simulink model "DPWM_VMC_lec22_r2017b"  (R2017b)
settings: Solver=FixedStepAuto  StartTime=0.0  StopTime=3e-3  FixedStep=Ts  RelTol=1e-3
PostLoadFcn:
  | , if any(exist('dsrtsu_mdlpostloadfcn', 'file') == [2, 3, 6]), try dsrtsu_mdlpostloadfcn('Execute', bdroot); catch fprintf('Error in PostLoadFcn (dsrtsu_mdlpostloadfcn) for model "%s":\n %s\n', bdroot, lasterr); end, end,
  | init_practical_voltage_source;
  | init_parameters;
InitFcn:
  | init_practical_voltage_source;
  | init_parameters;
values from neighbouring files (symbols this model uses):
  C = 200e-6    (= 0.0002)    [init_parameters.m]
  DCM_en = 0    [init_parameters.m]
  I0_final = 20    [init_parameters.m]
  I0_stepTime = 2.0e-3    (= 0.002)    [init_parameters.m]
  i_L_init = 1    [init_parameters.m]
  Kd = 0.5*C    (= 0.0001)    [init_parameters.m]
  Ki = 50000    [init_parameters.m]
  Kp = 10    [init_parameters.m]
  L = 0.5e-6    (= 5e-07)    [init_parameters.m]
  N = 1000    [init_parameters.m]
  R = 1    [init_parameters.m]
  r_C = 3e-3    (= 0.003)    [init_parameters.m]
  r_d = rds_on_sw2    (= 0.005)    [init_parameters.m]
  r_L = 5e-3    (= 0.005)    [init_parameters.m]
  rds_on_sw1 = 5e-3    (= 0.005)    [init_parameters.m]
  T_Vin_stepTime = 1.5e-3    (= 0.0015)    [init_parameters.m]
  Ts = 10e-9    (= 1e-08)    [init_parameters.m]
  Tsw = 2e-6    (= 2e-06)    [init_parameters.m]
  v_C_init = 1.1    [init_parameters.m]
  Vd = 0.55    [init_parameters.m]
  Vff = 1/Vin    (= 0.0833333333333)    [init_parameters.m]
  Vin = 12    [init_parameters.m]
  Vin_final = 0    [init_parameters.m]
  Vmax = 10    [init_parameters.m]
  Vref = 1.0    (= 1)    [init_parameters.m]
  Vref_final = 0    [init_parameters.m]
  Vref_stepTime = 2.2e-3    (= 0.0022)    [init_parameters.m]
libraries: simulink x5
Description:
  | Standard RTI1005 template.
  | Supported MATLAB version:  R2017b.
settings Model: Tag=RTI1005  DSRTSU_INTERNAL_RTI_VER=540  DSRTSU_INTERNAL_RTI_TYPE=rti1005  RTICANMMDATA=struct('GeneralSetupData',struct('modelroot','C:\Projects\Simulink\PE_2\w1\lec7','generalsettings',struct('filesettings',struct('destfolder',struct('Name','RTICANMM_FILES','Check',1),'buildfolder',struct('Name','.','Check',1),'AbsDestfolder',struct('Name','C:\Projects\Simulink\PE_2\w1\lec7\RTICANMM_FILES'),'AbsBuildfolder',struct('Name','C:\Projects\Simulink\PE_2\w1\lec7'))),'options',struct('addpaths',1,'rmpaths',1,'addtrcexclusion',logical(1),'cannavigator',struct('checkmonitoring',0),'show_usrtrc',0,'use_usrtrc',0),'advanced',struct('options',ones(1,100)),'MPSetup',{{}},'RTI',struct('Type','RTI1005','Ver','7.12','Date','02-May-2019'),'modelname','DPWM_VMC_lec21','block','DPWM_VMC_lec21'))  DSRTSU_INTERNAL_RTIFPGA=130  Creator=CA72672  LastModifiedBy=samee
settings SolverCC: ZeroCrossAlgorithm=Adaptive
settings OptimizationCC: BlockReduction=off  OptimizeBlockIOStorage=off  BufferReuse=off  GlobalBufferReuse=off  ExpressionFolding=off  LocalBlockOutputs=off
settings DebuggingCC: IgnoredZcDiagnostic=none
settings HardwareCC: ProdBitPerPointer=32  ProdBitPerSizeT=32  ProdBitPerPtrDiffT=32  ProdLargestAtomicInteger=Integer  ProdEndianess=BigEndian  ProdWordSize=32  ProdHWDeviceType=Custom Processor->Custom  TargetIntDivRoundTo=Zero  TargetEndianess=BigEndian  TargetHWDeviceType=Custom Processor->Custom
settings SFSimCC: MATLABDynamicMemAlloc=off
settings RTWCC: Description=dSPACE DS1005 Hardware Platform  SystemTargetFile=rti1005.tlc  MakeCommand=make_rti  TemplateMakefile=rti1005.tmf
settings CodeAppCC: StateflowObjectComments=on
settings STFCustomTargetCC: ParMdlRefBuildCompliant=on  MatFileLogging=on  GRTInterface=off  SystemTargetFile=rti1005.tlc
settings GRTTargetCC: TargetLangStandard=C89/C90 (ANSI)  CompOptLevelCompliant=off  ConcurrentExecutionCompliant=off  CombineOutputUpdateFcns=off  CPPClassGenCompliant=off  UseToolchainInfoCompliant=off
settings ConfigComp: CovMetricSettings=dswe

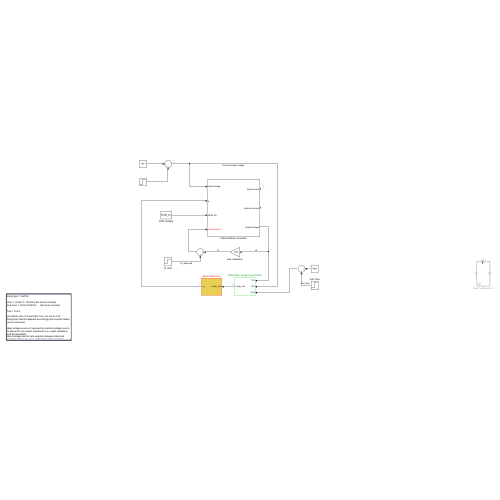
[thumbnail: Simulink's stored preview of the top-level diagram]
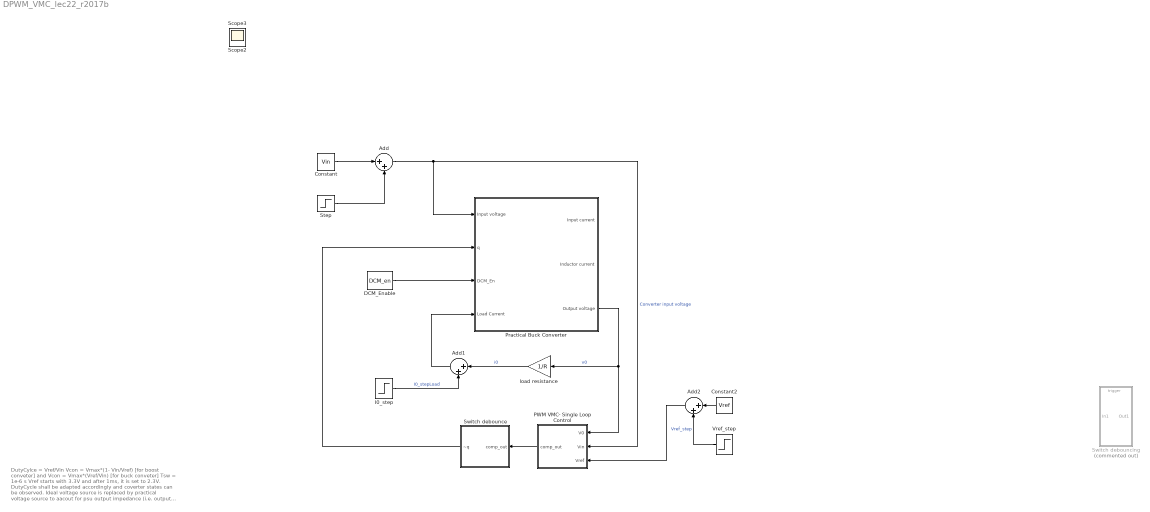
== system DPWM_VMC_lec22_r2017b ==
  note: DutyCylce = Vref/Vin
      |
      | Vcon = Vmax*(1- Vin/Vref)	[for boost conveter]
      | and Vcon = Vmax*(Vref/Vin)	[for buck conveter]
      |
      | Tsw = 1e-6 s
      |
      | Vref starts with 3.3V and after 1ms, it is set to 2.3V.
      | DutyCycle shall be adapted accordingly and coverter states can be observed.
      |
      | Ideal voltage source is replaced by practical voltage source to aacout for psu output impedance (i.e. output resistance and finit bandwidt)
      | Input voltage selector lets selection between ideal and practical voltage sources. -->Prameter in the script file: 'ideal_en'
  Add : Sum  Inputs=|++
  Add1 : Sum  Inputs=|++
  Add2 : Sum  Inputs=|++
  Constant : Constant  Value=Vin
  Constant2 : Constant  Value=Vref
  DCM_Enable : Constant  Value=DCM_en  OutDataTypeStr=boolean
  I0_step : Step  Time=I0_stepTime  After=I0_final  SampleTime=Ts
  PWM VMC- Single Loop Control : Subsystem
  Practical Buck Converter : Subsystem
  Step : Step  Time=T_Vin_stepTime  After=Vin_final  SampleTime=0
  Switch debounce : Subsystem
  Switch debouncing : Subsystem  Commented=on  TreatAsAtomicUnit=on
  Vref_step : Step  Time=Vref_stepTime  After=Vref_final  SampleTime=Ts
  load resistance : Gain  Gain=1/R
  Scope2 : Scope
  Scope3 : Scope
  wires:
  PWM VMC- Single Loop Control/1(comp_out) -> Switch debounce/1(comp_out)
  Constant/1 -> Add/1
  Step/1 -> Add/2
  Add/1 -> PWM VMC- Single Loop Control/2(Vin), Practical Buck Converter/1(Input voltage)  "Converter input voltage"
  DCM_Enable/1 -> Practical Buck Converter/3(DCM_En)
  I0_step/1 -> Add1/2  "I0_stepLoad"
  Practical Buck Converter/3(Output voltage) -> PWM VMC- Single Loop Control/1(V0), load resistance/1  "v0"
  Add1/1 -> Practical Buck Converter/4(Load Current)
  load resistance/1 -> Add1/1  "i0"
  Switch debounce/1(~q) -> Practical Buck Converter/2(q)
  Constant2/1 -> Add2/1
  Vref_step/1 -> Add2/2  "Vref_step"
  Add2/1 -> PWM VMC- Single Loop Control/3(Vref)

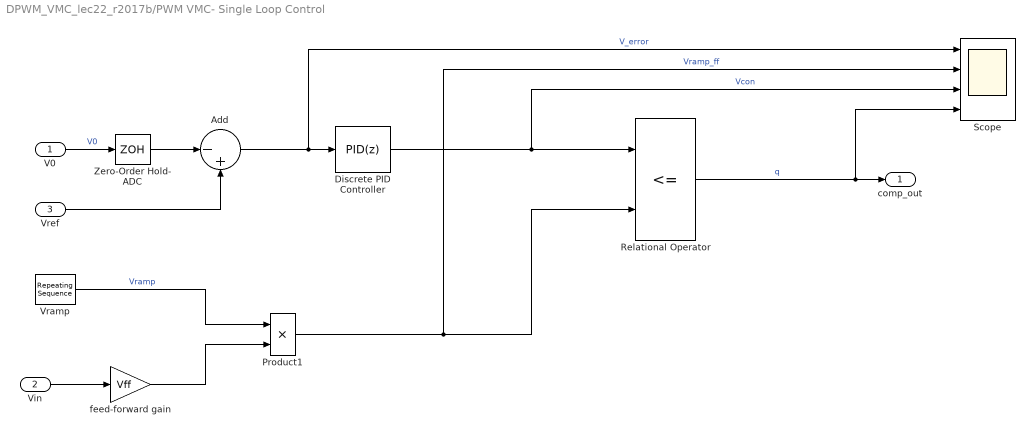
== system DPWM_VMC_lec22_r2017b/PWM VMC- Single Loop Control ==
  V0 : Inport
  Vin : Inport  Port=2
  Vref : Inport  Port=3
  Add : Sum  Inputs=|-+
  Discrete PID Controller : simulink/Continuous/PID Controller  Controller=PID  Form=Parallel  TimeDomain=Discrete-time  SampleTime=Ts  IntegratorMethod=Forward Euler  FilterMethod=Forward Euler  ControllerParametersSource=internal  P=Kp  I=Ki  D=Kd  N=N  UseFilter=off  TunerSelectOption=Transfer Function Based (PID Tuner App)  InitialConditionSource=internal  InitialConditionForIntegrator=0  InitialConditionForFilter=0  DifferentiatorICPrevScaledInput=0  ExternalReset=none  TrackingMode=off  Kt=1  LimitOutput=off  UpperSaturationLimit=inf  LowerSaturationLimit=-inf  LinearizeAsGain=off  AntiWindupMode=none  Kb=1  POutMin=[]  POutMax=[]  IOutMin=[]  IOutMax=[]  DOutMin=[]  DOutMax=[]  NOutMin=[]  NOutMax=[]  SumOutMin=[]  SumOutMax=[]  SaturationOutMin=[]  SaturationOutMax=[]  PParamMin=[]  PParamMax=[]  IParamMin=[]  IParamMax=[]  DParamMin=[]  DParamMax=[]  NParamMin=[]  NParamMax=[]  KbParamMin=[]  KbParamMax=[]  KtParamMin=[]  KtParamMax=[]  KbOutMin=[]  KbOutMax=[]  KtOutMin=[]  KtOutMax=[]  IntegratorOutMin=[]  IntegratorOutMax=[]  FilterOutMin=[]  FilterOutMax=[]  SumI1OutMin=[]  SumI1OutMax=[]  SumI2OutMin=[]  SumI2OutMax=[]  SumI3OutMin=[]  SumI3OutMax=[]  SumDOutMin=[]  SumDOutMax=[]  DifferentiatorOutMin=[]  DifferentiatorOutMax=[]  FilterDiffOutCoefMin=[]  FilterDiffOutCoefMax=[]  ReciprocalOutMin=[]  ReciprocalOutMax=[]  SumDenOutMin=[]  SumDenOutMax=[]  SumNumOutMin=[]  SumNumOutMax=[]  DivideOutMin=[]  DivideOutMax=[]  IntegratorContinuousStateAttributes=''  IntegratorStateMustResolveToSignalObject=off  IntegratorRTWStateStorageClass=Auto  FilterContinuousStateAttributes=''  FilterStateMustResolveToSignalObject=off  FilterRTWStateStorageClass=Auto  InitialConditionSetting=State (most efficient)
  Product1 : Product
  Relational Operator : RelationalOperator  Operator=<=  OutDataTypeStr=boolean  RndMeth=Simplest
  Scope : Scope  NumInputPorts=4
  Vramp : simulink/Sources/Repeating Sequence  rep_seq_t=[0 Tsw]  rep_seq_y=[0 Vmax]
  Zero-Order Hold- ADC : ZeroOrderHold  SampleTime=Tsw
  feed-forward gain : Gain  Gain=Vff
  comp_out : Outport  VectorParamsAs1DForOutWhenUnconnected=off
  wires:
  Discrete PID Controller/1 -> Scope/3, Relational Operator/1  "Vcon"
  Add/1 -> Scope/1, Discrete PID Controller/1  "V_error"
  Vin/1 -> feed-forward gain/1
  Vramp/1 -> Product1/1  "Vramp"
  feed-forward gain/1 -> Product1/2
  Relational Operator/1 -> Scope/4, comp_out/1  "q"
  V0/1 -> Zero-Order Hold- ADC/1  "V0"
  Vref/1 -> Add/2
  Product1/1 -> Relational Operator/2, Scope/2  "Vramp_ff"
  Zero-Order Hold- ADC/1 -> Add/1

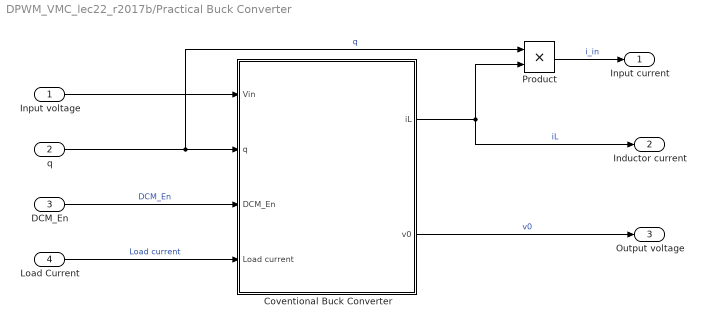
== system DPWM_VMC_lec22_r2017b/Practical Buck Converter ==
  Input voltage : Inport
  q : Inport  Port=2
  DCM_En : Inport  Port=3
  Load Current : Inport  Port=4
  Coventional Buck Converter : Subsystem
  Product : Product
  Input current : Outport  VectorParamsAs1DForOutWhenUnconnected=off
  Inductor current : Outport  Port=2  VectorParamsAs1DForOutWhenUnconnected=off
  Output voltage : Outport  Port=3  VectorParamsAs1DForOutWhenUnconnected=off
  wires:
  Input voltage/1 -> Coventional Buck Converter/1(Vin)
  DCM_En/1 -> Coventional Buck Converter/3(DCM_En)  "DCM_En"
  Load Current/1 -> Coventional Buck Converter/4(Load current)  "Load current"
  Coventional Buck Converter/1(iL) -> Inductor current/1, Product/2  "iL"
  Coventional Buck Converter/2(v0) -> Output voltage/1  "v0"
  q/1 -> Product/1, Coventional Buck Converter/2(q)  "q"
  Product/1 -> Input current/1  "i_in"

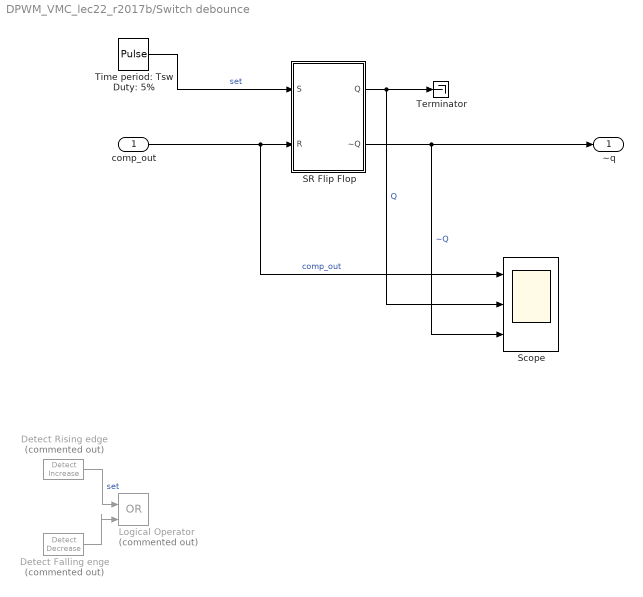
== system DPWM_VMC_lec22_r2017b/Switch debounce ==
  comp_out : Inport
  Detect Falling enge : simulink/Logic and Bit Operations/Detect Decrease  Commented=on  vinit=0.0  OutDataTypeStr=boolean
  Detect Rising edge : simulink/Logic and Bit Operations/Detect Increase  Commented=on  vinit=0.0  OutDataTypeStr=boolean
  Logical Operator : Logic  Commented=on  Operator=OR  IconShape=distinctive  AllPortsSameDT=off  OutDataTypeStr=boolean
  SR Flip Flop : Subsystem
  Scope : Scope  NumInputPorts=3
  Terminator : Terminator
  Time period: Tsw Duty: 5% : DiscretePulseGenerator  PulseType=Time based  Period=Tsw  PulseWidth=5
  ~q : Outport  VectorParamsAs1DForOutWhenUnconnected=off
  wires:
  SR Flip Flop/2(~Q) -> ~q/1, Scope/3  "~Q"
  SR Flip Flop/1(Q) -> Scope/2, Terminator/1  "Q"
  comp_out/1 -> Scope/1, SR Flip Flop/2(R)  "comp_out"
  Detect Falling enge/1 -> Logical Operator/2
  Detect Rising edge/1 -> Logical Operator/1  "set"
  Time period: Tsw Duty: 5%/1 -> SR Flip Flop/1(S)  "set"

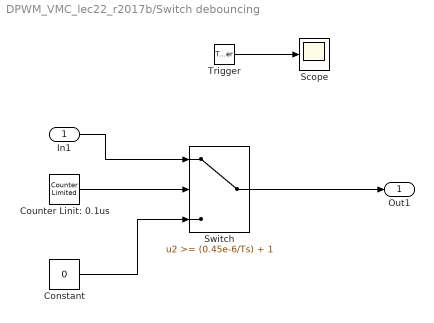
== system DPWM_VMC_lec22_r2017b/Switch debouncing ==
  In1 : Inport
  Trigger : TriggerPort  VariantControl=Variant  ShowOutputPort=on  PortDimensions=1
  Constant : Constant  Value=0
  Counter Linit: 0.1us : simulink/Sources/Counter Limited  uplimit=(0.45e-6/Ts) + 1  tsamp=-1
  Scope : Scope
  Switch : Switch  Threshold=(0.45e-6/Ts) + 1
  Out1 : Outport  VectorParamsAs1DForOutWhenUnconnected=off
  wires:
  In1/1 -> Switch/1
  Switch/1 -> Out1/1
  Counter Linit: 0.1us/1 -> Switch/2
  Constant/1 -> Switch/3
  Trigger/1 -> Scope/1

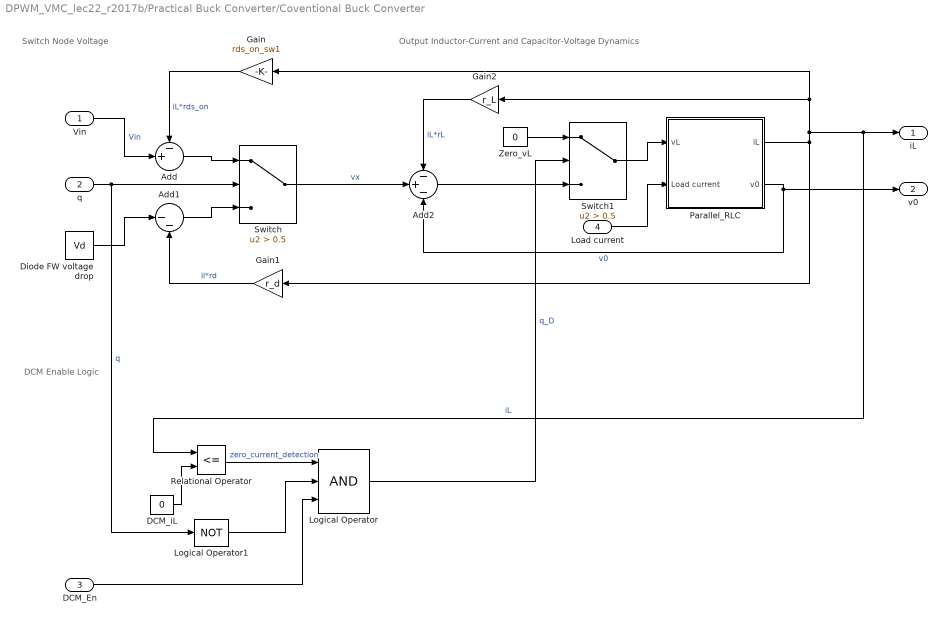
== system DPWM_VMC_lec22_r2017b/Practical Buck Converter/Coventional Buck Converter ==
  note: Switch Node Voltage
  note: Output Inductor-Current and
      | Capacitor-Voltage Dynamics
  note: DCM Enable Logic
  Vin : Inport
  q : Inport  Port=2
  DCM_En : Inport  Port=3
  Load current : Inport  Port=4
  Add : Sum  Inputs=-+|
  Add1 : Sum  Inputs=|--
  Add2 : Sum  Inputs=-+-
  DCM_iL : Constant  Value=0
  Diode FW voltage drop : Constant  Value=Vd
  Gain : Gain  Gain=rds_on_sw1
  Gain1 : Gain  Gain=r_d
  Gain2 : Gain  Gain=r_L
  Logical Operator : Logic  Inputs=3  IconShape=distinctive  AllPortsSameDT=off  OutDataTypeStr=boolean
  Logical Operator1 : Logic  Operator=NOT  Inputs=3  IconShape=distinctive  AllPortsSameDT=off  OutDataTypeStr=boolean
  Parallel_RLC : Subsystem
  Relational Operator : RelationalOperator  Operator=<=  OutDataTypeStr=boolean  RndMeth=Simplest
  Switch : Switch  Criteria=u2 > Threshold  Threshold=0.5
  Switch1 : Switch  Criteria=u2 > Threshold  Threshold=0.5
  Zero_vL : Constant  Value=0
  iL : Outport  VectorParamsAs1DForOutWhenUnconnected=off
  v0 : Outport  Port=2  VectorParamsAs1DForOutWhenUnconnected=off
  wires:
  Load current/1 -> Parallel_RLC/2(Load current)
  DCM_En/1 -> Logical Operator/3
  Logical Operator1/1 -> Logical Operator/2
  Relational Operator/1 -> Logical Operator/1  "zero_current_detection"
  DCM_iL/1 -> Relational Operator/2
  Zero_vL/1 -> Switch1/1
  Logical Operator/1 -> Switch1/2  "q_D"
  Switch1/1 -> Parallel_RLC/1(vL)
  Add2/1 -> Switch1/3
  Gain2/1 -> Add2/1  "iL*rL"
  Diode FW voltage drop/1 -> Add1/1
  Add1/1 -> Switch/3
  Switch/1 -> Add2/2  "vx"
  Gain1/1 -> Add1/2  "il*rd"
  Gain/1 -> Add/1  "iL*rds_on"
  Parallel_RLC/1(iL) -> Gain2/1, Gain/1, iL/1, Relational Operator/1, Gain1/1  "iL"
  Add/1 -> Switch/1
  Parallel_RLC/2(v0) -> v0/1, Add2/3  "v0"
  Vin/1 -> Add/2  "Vin"
  q/1 -> Logical Operator1/1, Switch/2  "q"

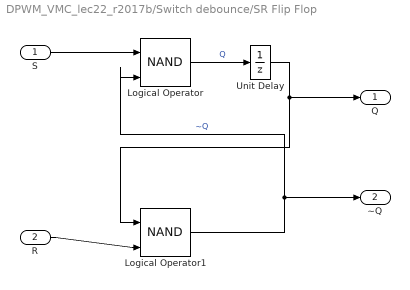
== system DPWM_VMC_lec22_r2017b/Switch debounce/SR Flip Flop ==
  S : Inport
  R : Inport  Port=2
  Logical Operator : Logic  Operator=NAND  IconShape=distinctive  AllPortsSameDT=off  OutDataTypeStr=boolean
  Logical Operator1 : Logic  Operator=NAND  IconShape=distinctive  AllPortsSameDT=off  OutDataTypeStr=boolean
  Unit Delay : UnitDelay  SampleTime=-1  HasFrameUpgradeWarning=on
  Q : Outport  VectorParamsAs1DForOutWhenUnconnected=off
  ~Q : Outport  Port=2  VectorParamsAs1DForOutWhenUnconnected=off
  wires:
  S/1 -> Logical Operator/1
  R/1 -> Logical Operator1/2
  Logical Operator/1 -> Unit Delay/1  "Q"
  Logical Operator1/1 -> ~Q/1, Logical Operator/2  "~Q"
  Unit Delay/1 -> Q/1, Logical Operator1/1

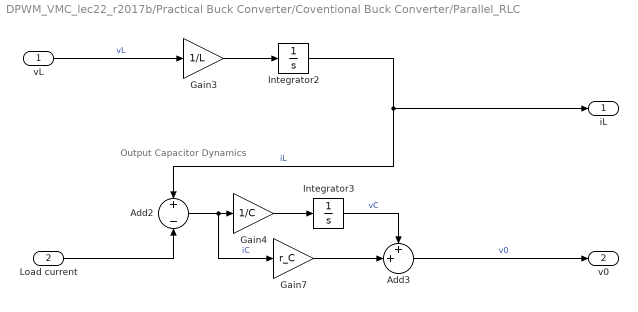
== system DPWM_VMC_lec22_r2017b/Practical Buck Converter/Coventional Buck Converter/Parallel_RLC ==
  note: Output Capacitor Dynamics
  vL : Inport
  Load current : Inport  Port=2
  Add2 : Sum  Inputs=+|-
  Add3 : Sum  Inputs=++|
  Gain3 : Gain  Gain=1/L
  Gain4 : Gain  Gain=1/C
  Gain7 : Gain  Gain=r_C
  Integrator2 : Integrator  InitialCondition=i_L_init
  Integrator3 : Integrator  InitialCondition=v_C_init
  iL : Outport  VectorParamsAs1DForOutWhenUnconnected=off
  v0 : Outport  Port=2  VectorParamsAs1DForOutWhenUnconnected=off
  wires:
  Add3/1 -> v0/1  "v0"
  Gain7/1 -> Add3/2
  Integrator3/1 -> Add3/1  "vC"
  Add2/1 -> Gain4/1, Gain7/1  "iC"
  Gain4/1 -> Integrator3/1
  Integrator2/1 -> iL/1, Add2/1  "iL"
  Gain3/1 -> Integrator2/1
  vL/1 -> Gain3/1  "vL"
  Load current/1 -> Add2/2
